simulink model "Modelo_MI_simulink_standalone_ver2020b"  (R2020b)
settings: Solver=ode5  StartTime=0.0  StopTime=tsim  FixedStep=tstep  MaxStep=1e-4  RelTol=1e-3
PreLoadFcn:
  | % Estructura para parametros del motor de induccion
  | 
  | inversor_select = 0;
  | tsim = 20;
  | tstep = 1e-4;
  | 
  | nomvals = struct('Pnom',745.7,'v_Srmsnom',230,'i_Srmsnom',0,'psi_Rmagnom',0,'w_Rnom',180.64,'tau_Rnom',0);
  | elecparams = struct('n_p',2,'R_S',2.516,'R_R',1.941,'L_S',0.234,'L_R',0.2303,'M',0.2226,'sigma',0,'gamma',0);
  | mechparams = struct('J',0.0062764,'b',0.00011);
  | 
  | nomvals.i_Srmsnom = nomvals.Pnom/nomvals.v_Srmsnom;
  | nomvals.psi_Rmagnom = elecparams.M*nomvals.i_Srmsnom/sqrt(2);
  | nomvals.tau_Rnom = nomvals.Pnom/nomvals.w_Rnom;
  | 
  | elecparams.sigma = elecparams.L_S-(elecparams.M^2/elecparams.L_R);
  | elecparams.gamma = (elecparams.R_S*elecparams.L_R^2+elecparams.R_R*elecparams.M^2)/(elecparams.sigma*elecparams.L_R^2);
  | 
  | MI_params = struct('nomvals',nomvals,'elecparams',elecparams,'mechparams',mechparams);
  | 
  | MI_bus_info = Simulink.Bus.createObject(MI_params);
  | MI_bus = evalin('base', MI_bus_info.busName);
libraries: powerlib x16, mcbcontrolslib x4, powerlib_meascontrol x2, simulink x1
settings Model: Creator=HP  LastModifiedBy=HP
settings DebuggingCC: UnconnectedInputMsg=none  UnconnectedOutputMsg=none  UnconnectedLineMsg=none
settings ModelReferenceCC: EnableRefExpFcnMdlSchedulingChecks=off

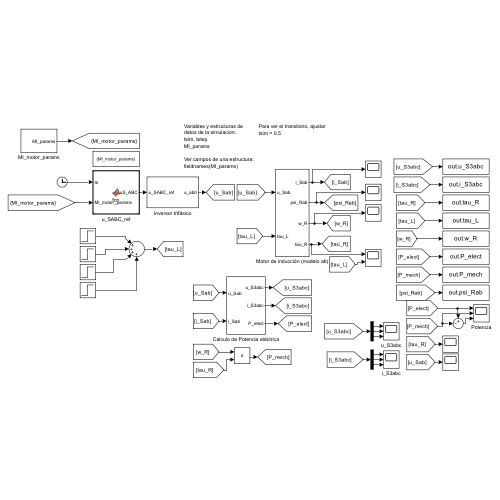
[thumbnail: Simulink's stored preview of the top-level diagram]
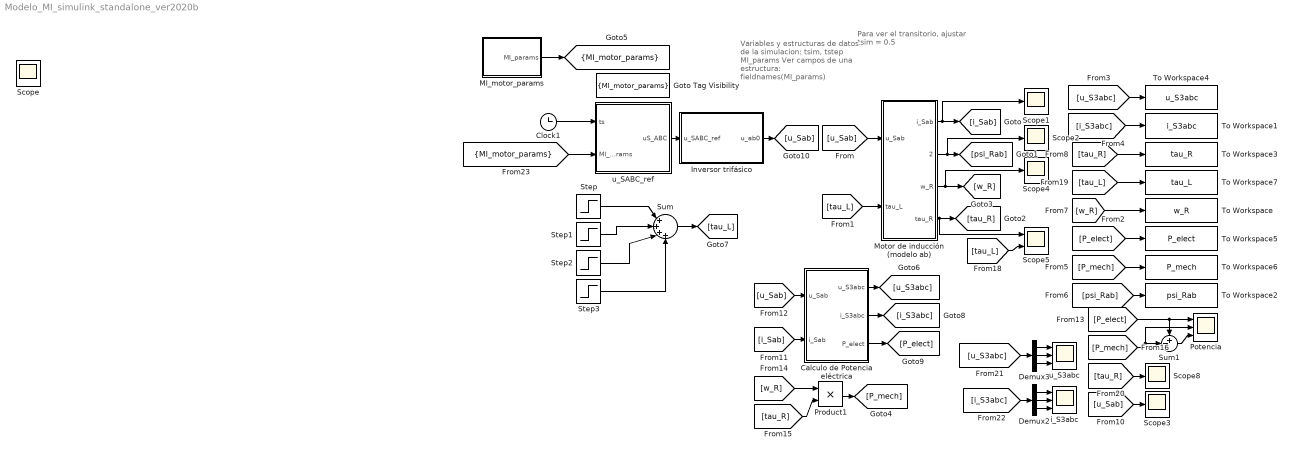
== system Modelo_MI_simulink_standalone_ver2020b ==
  note: Para ver el transitorio, ajustar
      | tsim = 0.5
  note: Variables y estructuras de datos de la simulacion:
      | tsim, tstep
      | MI_params
      |
      | Ver campos de una estructura:
      | fieldnames(MI_params)
  Calculo de Potencia eléctrica : Subsystem
  Clock1 : Clock
  Demux2 : Demux  Outputs=3
  Demux3 : Demux  Outputs=3
  Goto Tag Visibility : GotoTagVisibility  GotoTag=MI_motor_params
  Inversor trifásico : Subsystem
  MI_motor_params : Subsystem
  Motor de inducción (modelo ab) : Subsystem
  Potencia : Scope  NumInputPorts=3
  Product1 : Product
  Scope{,1..4,8} (6 alike) : Scope
  Scope5 : Scope  NumInputPorts=2
  Step : Step  Time=2  After=MI_params.nomvals.tau_Rnom/4  SampleTime=0
  Step1 : Step  Time=4  After=MI_params.nomvals.tau_Rnom/4  SampleTime=0
  Step2 : Step  Time=6  After=MI_params.nomvals.tau_Rnom/4  SampleTime=0
  Step3 : Step  Time=8  After=MI_params.nomvals.tau_Rnom/4  SampleTime=0
  Sum : Sum  Inputs=|++++
  Sum1 : Sum  Inputs=+-|
  To Workspace : ToWorkspace  VariableName=w_R  SaveFormat=Timeseries  SampleTime=-1
  To Workspace1 : ToWorkspace  VariableName=i_S3abc  SaveFormat=Timeseries  SampleTime=-1
  To Workspace2 : ToWorkspace  VariableName=psi_Rab  SaveFormat=Timeseries  SampleTime=-1
  To Workspace3 : ToWorkspace  VariableName=tau_R  SaveFormat=Timeseries  SampleTime=-1
  To Workspace4 : ToWorkspace  VariableName=u_S3abc  SaveFormat=Timeseries  SampleTime=-1
  To Workspace5 : ToWorkspace  VariableName=P_elect  SaveFormat=Timeseries  SampleTime=-1
  To Workspace6 : ToWorkspace  VariableName=P_mech  SaveFormat=Timeseries  SampleTime=-1
  To Workspace7 : ToWorkspace  VariableName=tau_L  SaveFormat=Timeseries  SampleTime=-1
  i_S3abc : Scope  NumInputPorts=3
  u_S3abc : Scope  NumInputPorts=3
  u_SABC_ref : MATLAB Function  TreatAsAtomicUnit=on
  tag scope: MI_motor_params=scoped
  wires:
  [w_R] -> To Workspace/1
  [i_S3abc] -> To Workspace1/1
  [tau_R] -> To Workspace3/1
  Step/1 -> Sum/1
  Step1/1 -> Sum/2
  Step2/1 -> Sum/3
  Step3/1 -> Sum/4
  Sum/1 -> [tau_L]
  [i_Sab] -> Calculo de Potencia eléctrica/2(i_Sab)
  Calculo de Potencia eléctrica/3(P_elect) -> [P_elect]
  Calculo de Potencia eléctrica/1(u_S3abc) -> [u_S3abc]
  [u_Sab] -> Calculo de Potencia eléctrica/1(u_Sab)
  Calculo de Potencia eléctrica/2(i_S3abc) -> [i_S3abc]
  [tau_L] -> Scope5/2
  Motor de inducción (modelo ab)/2(psi_Rab) -> Scope2/1, [psi_Rab]
  Motor de inducción (modelo ab)/1(i_Sab) -> Scope1/1, [i_Sab]
  Motor de inducción (modelo ab)/4(tau_R) -> Scope5/1, [tau_R]
  Motor de inducción (modelo ab)/3(w_R) -> [w_R], Scope4/1
  [u_Sab] -> Motor de inducción (modelo ab)/1(u_Sab)
  [tau_L] -> Motor de inducción (modelo ab)/2(tau_L)
  [u_S3abc] -> To Workspace4/1
  Demux3/3 -> u_S3abc/3
  Demux2/3 -> i_S3abc/3
  Demux3/1 -> u_S3abc/1
  Demux2/1 -> i_S3abc/1
  Demux3/2 -> u_S3abc/2
  Demux2/2 -> i_S3abc/2
  [P_elect] -> To Workspace5/1
  [P_mech] -> To Workspace6/1
  [tau_L] -> To Workspace7/1
  [MI_motor_params] -> u_SABC_ref/2(MI_motor_params)
  Clock1/1 -> u_SABC_ref/1(ts)
  [psi_Rab] -> To Workspace2/1
  [u_Sab] -> Scope3/1
  u_SABC_ref/1(uS_ABC) -> Inversor trifásico/1(u_SABC_ref)
  Inversor trifásico/1(u_ab0) -> [u_Sab]
  [tau_R] -> Scope8/1
  [P_elect] -> Potencia/1, Sum1/1
  [tau_R] -> Product1/2
  [P_mech] -> Potencia/2, Sum1/2
  Product1/1 -> [P_mech]
  Sum1/1 -> Potencia/3
  [w_R] -> Product1/1
  [u_S3abc] -> Demux3/1
  [i_S3abc] -> Demux2/1
  MI_motor_params/1(MI_params) -> [MI_motor_params]

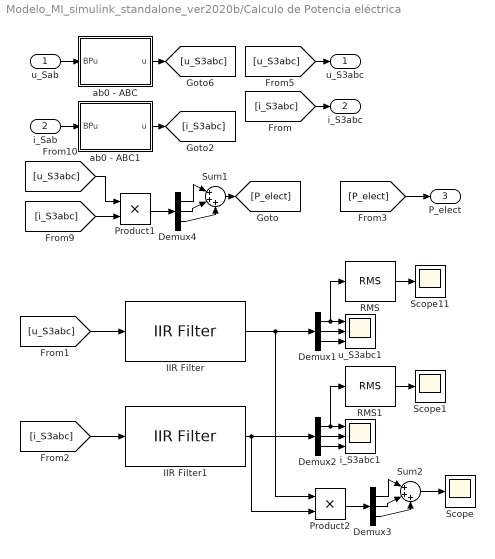
== system Modelo_MI_simulink_standalone_ver2020b/Calculo de Potencia eléctrica ==
  u_Sab : Inport
  i_Sab : Inport  Port=2
  Demux{1..4} (4 alike) : Demux  Outputs=3
  IIR Filter : mcbcontrolslib/IIR Filter  VariantControl=Low Pass Filter  VariantSelect=Low-pass  Filter_constant=0.04  advancedSettings=on  Ts=50e-6  cutOff_freq=132.6291
  IIR Filter1 : mcbcontrolslib/IIR Filter  VariantControl=Low Pass Filter  VariantSelect=Low-pass  Filter_constant=0.04  advancedSettings=on  Ts=50e-6  cutOff_freq=132.6291
  Product1 : Product
  Product2 : Product
  RMS : powerlib_meascontrol/Measurements/RMS  TrueRMS=on  Freq=60  RMSInit=120  Ts=0
  RMS1 : powerlib_meascontrol/Measurements/RMS  TrueRMS=on  Freq=60  RMSInit=120  Ts=0
  Scope : Scope
  Scope1 : Scope
  Scope11 : Scope
  Sum1 : Sum  Inputs=|+++
  Sum2 : Sum  Inputs=|+++
  ab0 - ABC : MATLAB Function  TreatAsAtomicUnit=on
  ab0 - ABC1 : MATLAB Function  TreatAsAtomicUnit=on
  i_S3abc1 : Scope  NumInputPorts=3
  u_S3abc1 : Scope  NumInputPorts=3
  u_S3abc : Outport
  i_S3abc : Outport  Port=2
  P_elect : Outport  Port=3
  wires:
  Demux4/1 -> Sum1/1
  [i_S3abc] -> Product1/2
  i_Sab/1 -> ab0 - ABC1/1(BPu)
  Demux4/3 -> Sum1/3
  [u_S3abc] -> Product1/1
  Demux4/2 -> Sum1/2
  Product1/1 -> Demux4/1
  u_Sab/1 -> ab0 - ABC/1(BPu)
  [u_S3abc] -> u_S3abc/1
  [i_S3abc] -> i_S3abc/1
  ab0 - ABC/1(u) -> [u_S3abc]
  ab0 - ABC1/1(u) -> [i_S3abc]
  IIR Filter/1 -> Product2/1, Demux1/1
  RMS/1 -> Scope11/1
  Demux1/2 -> u_S3abc1/2
  Demux1/3 -> u_S3abc1/3
  Demux1/1 -> RMS/1, u_S3abc1/1
  [u_S3abc] -> IIR Filter/1
  Demux2/1 -> RMS1/1, i_S3abc1/1
  RMS1/1 -> Scope1/1
  Demux2/2 -> i_S3abc1/2
  IIR Filter1/1 -> Product2/2, Demux2/1
  [i_S3abc] -> IIR Filter1/1
  Demux2/3 -> i_S3abc1/3
  Demux3/2 -> Sum2/2
  Demux3/3 -> Sum2/3
  Sum2/1 -> Scope/1
  Product2/1 -> Demux3/1
  Demux3/1 -> Sum2/1
  Sum1/1 -> [P_elect]
  [P_elect] -> P_elect/1

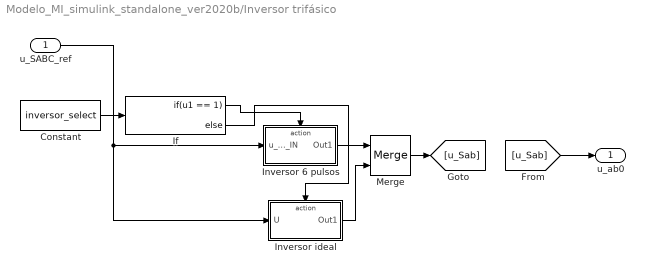
== system Modelo_MI_simulink_standalone_ver2020b/Inversor trifásico ==
  u_SABC_ref : Inport
  Constant : Constant  Value=inversor_select
  If : If  IfExpression=u1 == 1
  Inversor 6 pulsos : Subsystem  TreatAsAtomicUnit=on
  Inversor ideal : Subsystem  TreatAsAtomicUnit=on
  Merge : Merge
  u_ab0 : Outport
  wires:
  [u_Sab] -> u_ab0/1
  If/1 -> Inversor 6 pulsos/Action
  If/2 -> Inversor ideal/Action
  Inversor 6 pulsos/1(Out1) -> Merge/1
  Inversor ideal/1(Out1) -> Merge/2
  Merge/1 -> [u_Sab]
  Constant/1 -> If/1
  u_SABC_ref/1 -> Inversor ideal/1(U), Inversor 6 pulsos/1(u_SABC_IN)

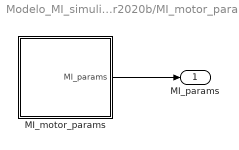
== system Modelo_MI_simulink_standalone_ver2020b/MI_motor_params ==
  MI_motor_params : MATLAB Function  TreatAsAtomicUnit=on
  MI_params : Outport
  wires:
  MI_motor_params/1(MI_params) -> MI_params/1

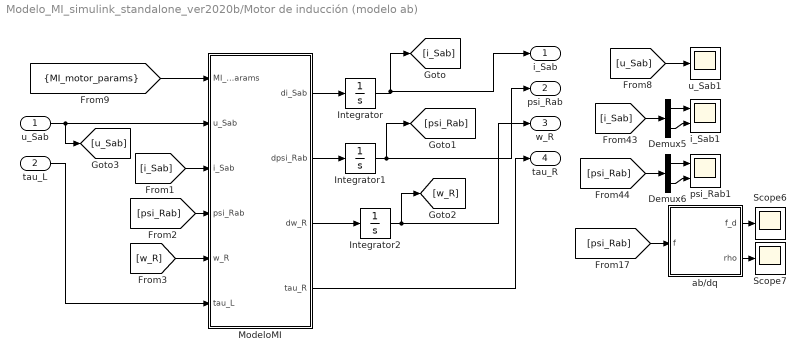
== system Modelo_MI_simulink_standalone_ver2020b/Motor de inducción (modelo ab) ==
  u_Sab : Inport
  tau_L : Inport  Port=2
  Demux5 : Demux  Outputs=2
  Demux6 : Demux  Outputs=2
  Integrator : Integrator
  Integrator1 : Integrator
  Integrator2 : Integrator
  ModeloMI : MATLAB Function  TreatAsAtomicUnit=on
  Scope6 : Scope
  Scope7 : Scope
  ab/dq : MATLAB Function  TreatAsAtomicUnit=on
  i_Sab1 : Scope  NumInputPorts=2
  psi_Rab1 : Scope  NumInputPorts=2
  u_Sab1 : Scope
  i_Sab : Outport
  psi_Rab : Outport  Port=2
  w_R : Outport  Port=3
  tau_R : Outport  Port=4
  wires:
  ModeloMI/3(dw_R) -> Integrator2/1
  [i_Sab] -> ModeloMI/3(i_Sab)
  [MI_motor_params] -> ModeloMI/1(MI_motor_params)
  [psi_Rab] -> ModeloMI/4(psi_Rab)
  [w_R] -> ModeloMI/5(w_R)
  Integrator2/1 -> w_R/1, [w_R]
  ModeloMI/2(dpsi_Rab) -> Integrator1/1
  tau_L/1 -> ModeloMI/6(tau_L)
  ModeloMI/1(di_Sab) -> Integrator/1
  u_Sab/1 -> ModeloMI/2(u_Sab), [u_Sab]
  ModeloMI/4(tau_R) -> tau_R/1
  Integrator/1 -> [i_Sab], i_Sab/1
  Integrator1/1 -> [psi_Rab], psi_Rab/1
  [psi_Rab] -> ab/dq/1(f)
  ab/dq/2(rho) -> Scope7/1
  Demux6/2 -> psi_Rab1/2
  Demux5/2 -> i_Sab1/2
  [u_Sab] -> u_Sab1/1
  Demux6/1 -> psi_Rab1/1
  [psi_Rab] -> Demux6/1
  Demux5/1 -> i_Sab1/1
  [i_Sab] -> Demux5/1
  ab/dq/1(f_d) -> Scope6/1

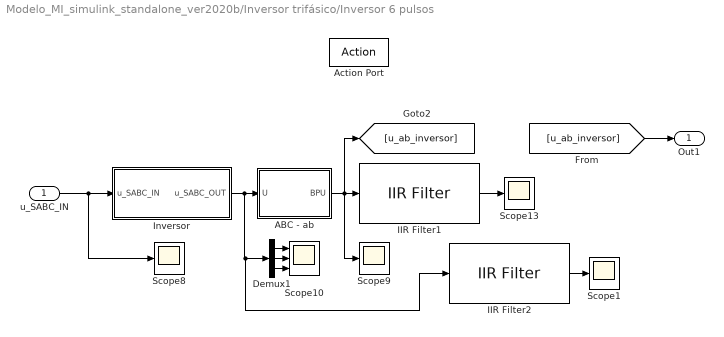
== system Modelo_MI_simulink_standalone_ver2020b/Inversor trifásico/Inversor 6 pulsos ==
  u_SABC_IN : Inport
  Action Port : ActionPort  ActionPortLabel=if(u1 == 1)
  ABC - ab : MATLAB Function  TreatAsAtomicUnit=on
  Demux1 : Demux  Outputs=3
  IIR Filter1 : mcbcontrolslib/IIR Filter  VariantControl=Low Pass Filter  VariantSelect=Low-pass  Filter_constant=0.04  advancedSettings=on  Ts=50e-6  cutOff_freq=132.6291
  IIR Filter2 : mcbcontrolslib/IIR Filter  VariantControl=Low Pass Filter  VariantSelect=Low-pass  Filter_constant=0.04  advancedSettings=on  Ts=50e-6  cutOff_freq=132.6291
  Inversor : Subsystem
  Scope{1,8..9,13} (4 alike) : Scope
  Scope10 : Scope  NumInputPorts=3
  Out1 : Outport
  wires:
  IIR Filter2/1 -> Scope1/1
  ABC - ab/1(BPU) -> [u_ab_inversor], IIR Filter1/1, Scope9/1
  Demux1/3 -> Scope10/3
  Inversor/1(u_SABC_OUT) -> IIR Filter2/1, Demux1/1, ABC - ab/1(U)
  Demux1/1 -> Scope10/1
  Demux1/2 -> Scope10/2
  IIR Filter1/1 -> Scope13/1
  u_SABC_IN/1 -> Scope8/1, Inversor/1(u_SABC_IN)
  [u_ab_inversor] -> Out1/1

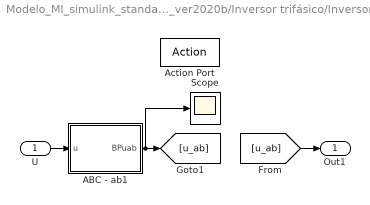
== system Modelo_MI_simulink_standalone_ver2020b/Inversor trifásico/Inversor ideal ==
  U : Inport
  Action Port : ActionPort  ActionPortLabel=else
  ABC - ab1 : MATLAB Function  TreatAsAtomicUnit=on
  Scope : Scope
  Out1 : Outport
  wires:
  ABC - ab1/1(BPuab) -> Scope/1, [u_ab]
  U/1 -> ABC - ab1/1(u)
  [u_ab] -> Out1/1

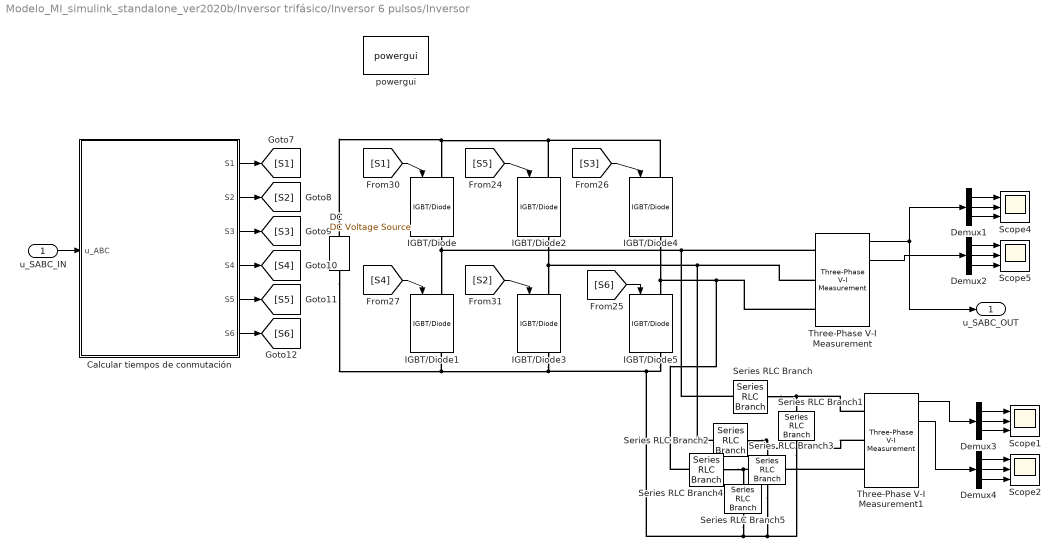
== system Modelo_MI_simulink_standalone_ver2020b/Inversor trifásico/Inversor 6 pulsos/Inversor ==
  u_SABC_IN : Inport
  Calcular tiempos de conmutación : Subsystem
  "DC " : powerlib/Electrical Sources/DC Voltage Source  Amplitude=310  Measurements=None
  Demux{1..4} (4 alike) : Demux  Outputs=3
  IGBT/Diode{,1..5} (6 alike) : powerlib/Power Electronics/IGBT//Diode  Ron=1e-3  Rs=1e5  Cs=inf  Measurements=on
  Scope{1..2,4..5} (4 alike) : Scope  NumInputPorts=3
  Series RLC Branch : powerlib/Elements/Series RLC Branch  LConnTagsString=__new0  RConnTagsString=__new0  BranchType=R  Resistance=1  Inductance=1e-3  SetiL0=off  InitialCurrent=0  Capacitance=1e-6  Setx0=off  InitialVoltage=0  Measurements=None
  Series RLC Branch1 : powerlib/Elements/Series RLC Branch  LConnTagsString=__new0  RConnTagsString=__new0  BranchType=C  Resistance=1  Inductance=1e-3  SetiL0=off  InitialCurrent=0  Capacitance=120e-6  Setx0=off  InitialVoltage=0  Measurements=None
  Series RLC Branch2 : powerlib/Elements/Series RLC Branch  LConnTagsString=__new0  RConnTagsString=__new0  BranchType=R  Resistance=1  Inductance=1e-3  SetiL0=off  InitialCurrent=0  Capacitance=1e-6  Setx0=off  InitialVoltage=0  Measurements=None
  Series RLC Branch3 : powerlib/Elements/Series RLC Branch  LConnTagsString=__new0  RConnTagsString=__new0  BranchType=C  Resistance=1  Inductance=1e-3  SetiL0=off  InitialCurrent=0  Capacitance=120e-6  Setx0=off  InitialVoltage=0  Measurements=None
  Series RLC Branch4 : powerlib/Elements/Series RLC Branch  LConnTagsString=__new0  RConnTagsString=__new0  BranchType=R  Resistance=1  Inductance=1e-3  SetiL0=off  InitialCurrent=0  Capacitance=1e-6  Setx0=off  InitialVoltage=0  Measurements=None
  Series RLC Branch5 : powerlib/Elements/Series RLC Branch  LConnTagsString=__new0  RConnTagsString=__new0  BranchType=C  Resistance=1  Inductance=1e-3  SetiL0=off  InitialCurrent=0  Capacitance=120e-6  Setx0=off  InitialVoltage=0  Measurements=None
  Three-Phase V-I Measurement : powerlib/Measurements/Three-Phase V-I Measurement  VoltageMeasurement=phase-to-phase  SetLabelV=off  LabelV=Vabc  Vpu=off  VpuLL=off  CurrentMeasurement=yes  SetLabelI=off  LabelI=Iabc  Ipu=off  Pbase=100e6  Vbase=500e3  OutputType=Complex  PhasorSimulation=off  PSBequivalent=0
  Three-Phase V-I Measurement1 : powerlib/Measurements/Three-Phase V-I Measurement  VoltageMeasurement=phase-to-phase  SetLabelV=off  LabelV=Vabc  Vpu=off  VpuLL=off  CurrentMeasurement=yes  SetLabelI=off  LabelI=Iabc  Ipu=off  Pbase=100e6  Vbase=500e3  OutputType=Complex  PhasorSimulation=off  PSBequivalent=0
  powergui : powerlib/powergui  Priority=1  SimulationMode=Continuous  SampleTime=10e-6  frequency=60  Iterations=50  frequencyindice=0  Pbase=100e6  ErrMax=1e-4  UnitsV=kV  UnitsW=MW  buscounter=0  FunctionMessages=off  echomessages=off  EnableUseOfTLC=off  CurrentSourceSwitches=on  DisableSnubberDevices=off  DisableRonSwitches=off  DisableVfSwitches=off  DisplayEquations=off  AutomaticDiscreteSolvers=off  SolverType=Tustin/Backward Euler (TBE)  Interpol=off  ExternalGateDelay=off  methode=off  Ts=10  x0status=blocks  SPID=off  SwTol=0  HookPort=off  NonlinearTolerance=1e-4  nMaxIteration=100  ContinueOnMaxIteration=off  RestoreLinks=warning  ResistiveCurrentMeasurement=off  Frange=[0:2:500]  Ylog=off  Xlog=on  ShowGrid=off  save=off  variable=ZData  structure=ScopeData1  ZoomFFT=off  StartTime=0.0  cycles=1  DisplayStyle=1  fundamental=50  FreqAxis=off  MaxFrequency=1000  frequencyindicesteady=1  RmsSteady=1  display=off
  u_SABC_OUT : Outport
  wires:
  [S5] -> IGBT/Diode2/1
  Demux2/3 -> Scope5/3
  Demux2/2 -> Scope5/2
  Three-Phase V-I Measurement/1 -> Demux1/1, u_SABC_OUT/1
  Demux1/2 -> Scope4/2
  Demux2/1 -> Scope5/1
  Demux1/1 -> Scope4/1
  Calcular tiempos de conmutación/5(S5) -> [S5]
  Three-Phase V-I Measurement/2 -> Demux2/1
  u_SABC_IN/1 -> Calcular tiempos de conmutación/1(u_ABC)
  [S3] -> IGBT/Diode4/1
  Calcular tiempos de conmutación/2(S2) -> [S2]
  Calcular tiempos de conmutación/6(S6) -> [S6]
  Calcular tiempos de conmutación/4(S4) -> [S4]
  [S1] -> IGBT/Diode/1
  Calcular tiempos de conmutación/3(S3) -> [S3]
  Calcular tiempos de conmutación/1(S1) -> [S1]
  Demux1/3 -> Scope4/3
  [S2] -> IGBT/Diode3/1
  [S6] -> IGBT/Diode5/1
  [S4] -> IGBT/Diode1/1
  Three-Phase V-I Measurement1/2 -> Demux4/1
  Three-Phase V-I Measurement1/1 -> Demux3/1
  Demux4/1 -> Scope2/1
  Demux3/1 -> Scope1/1
  Demux4/2 -> Scope2/2
  Demux3/3 -> Scope1/3
  Demux3/2 -> Scope1/2
  Demux4/3 -> Scope2/3
  connections:
  IGBT/Diode5/LConn1 -- Series RLC Branch4/LConn1 -- Three-Phase V-I Measurement/LConn3 -- IGBT/Diode4/RConn1
  IGBT/Diode2/RConn1 -- Three-Phase V-I Measurement/LConn2 -- Series RLC Branch2/LConn1 -- IGBT/Diode3/LConn1
  "DC "/RConn1 -- IGBT/Diode/LConn1 -- IGBT/Diode4/LConn1 -- IGBT/Diode2/LConn1
  IGBT/Diode/RConn1 -- Series RLC Branch/LConn1 -- Three-Phase V-I Measurement/LConn1 -- IGBT/Diode1/LConn1
  Series RLC Branch/RConn1 -- Three-Phase V-I Measurement1/LConn1 -- Series RLC Branch1/LConn1
  IGBT/Diode3/RConn1 -- Series RLC Branch1/RConn1 -- Series RLC Branch3/RConn1 -- Series RLC Branch5/RConn1 -- IGBT/Diode5/RConn1 -- "DC "/LConn1 -- IGBT/Diode1/RConn1
  Series RLC Branch2/RConn1 -- Three-Phase V-I Measurement1/LConn2 -- Series RLC Branch3/LConn1
  Series RLC Branch4/RConn1 -- Three-Phase V-I Measurement1/LConn3 -- Series RLC Branch5/LConn1

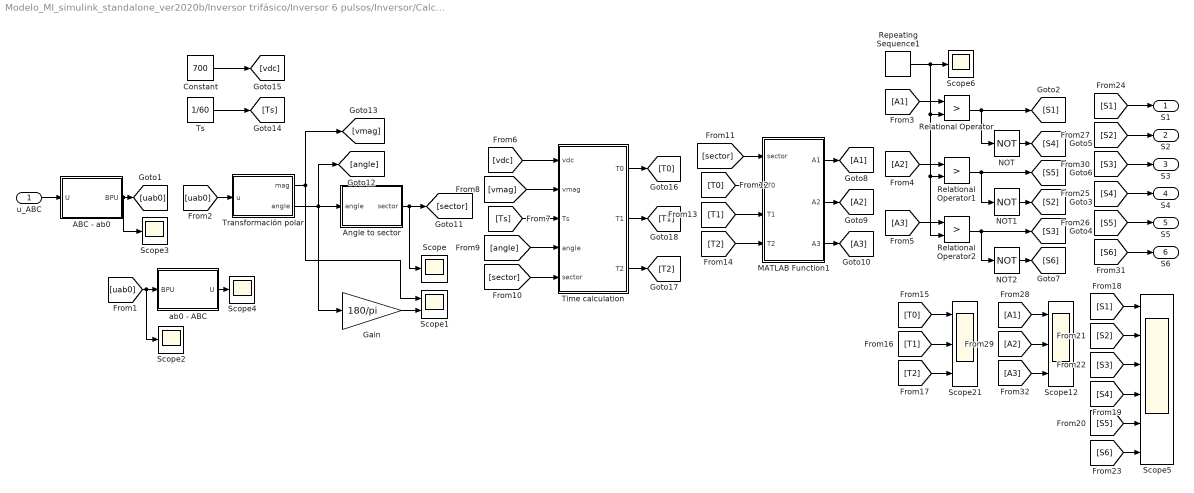
== system Modelo_MI_simulink_standalone_ver2020b/Inversor trifásico/Inversor 6 pulsos/Inversor/Calcular tiempos de conmutación ==
  u_ABC : Inport
  ABC - ab0 : MATLAB Function  TreatAsAtomicUnit=on
  Angle to sector : MATLAB Function  TreatAsAtomicUnit=on
  Constant : Constant  Value=700
  Gain : Gain  Gain=180/pi
  MATLAB Function1 : MATLAB Function  TreatAsAtomicUnit=on
  NOT : Logic  Operator=NOT  IconShape=distinctive  AllPortsSameDT=off  OutDataTypeStr=boolean
  NOT1 : Logic  Operator=NOT  IconShape=distinctive  AllPortsSameDT=off  OutDataTypeStr=boolean
  NOT2 : Logic  Operator=NOT  IconShape=distinctive  AllPortsSameDT=off  OutDataTypeStr=boolean
  Relational Operator : RelationalOperator  Operator=>  OutDataTypeStr=boolean  RndMeth=Nearest
  Relational Operator1 : RelationalOperator  Operator=>  OutDataTypeStr=boolean  RndMeth=Nearest
  Relational Operator2 : RelationalOperator  Operator=>  OutDataTypeStr=boolean  RndMeth=Nearest
  Repeating Sequence1 : simulink/Sources/Repeating Sequence  rep_seq_t=[0 1]*[1/5000]  rep_seq_y=[0 1/60]
  Scope{,2..4,6} (5 alike) : Scope
  Scope1 : Scope  NumInputPorts=2
  Scope12 : Scope  NumInputPorts=3
  Scope21 : Scope  NumInputPorts=3
  Scope5 : Scope  NumInputPorts=6
  Time calculation : MATLAB Function  TreatAsAtomicUnit=on
  Transformación polar : MATLAB Function  TreatAsAtomicUnit=on
  Ts : Constant  Value=1/60
  ab0 - ABC : MATLAB Function  TreatAsAtomicUnit=on
  S1 : Outport
  S2 : Outport  Port=2
  S3 : Outport  Port=3
  S4 : Outport  Port=4
  S5 : Outport  Port=5
  S6 : Outport  Port=6
  wires:
  [vmag] -> Time calculation/2(vmag)
  [sector] -> Time calculation/5(sector)
  Relational Operator2/1 -> NOT2/1, [S3]
  [Ts] -> Time calculation/3(Ts)
  NOT2/1 -> [S6]
  [S6] -> Scope5/6
  Transformación polar/1(mag) -> [vmag], Scope1/1
  [T1] -> Scope21/2
  [S3] -> Scope5/3
  Time calculation/3(T2) -> [T2]
  [T2] -> Scope21/3
  [T1] -> MATLAB Function1/3(T1)
  [uab0] -> Transformación polar/1(u)
  Time calculation/2(T1) -> [T1]
  Relational Operator1/1 -> NOT1/1, [S5]
  NOT1/1 -> [S2]
  Angle to sector/1(sector) -> [sector], Scope/1
  [S1] -> Scope5/1
  [uab0] -> Scope2/1, ab0 - ABC/1(BPU)
  [angle] -> Time calculation/4(angle)
  [S4] -> Scope5/4
  [A2] -> Relational Operator1/1
  MATLAB Function1/2(A2) -> [A2]
  NOT/1 -> [S4]
  [T2] -> MATLAB Function1/4(T2)
  Transformación polar/2(angle) -> [angle], Gain/1, Angle to sector/1(angle)
  MATLAB Function1/1(A1) -> [A1]
  Gain/1 -> Scope1/2
  Relational Operator/1 -> NOT/1, [S1]
  [A3] -> Scope12/3
  ab0 - ABC/1(U) -> Scope4/1
  Repeating Sequence1/1 -> Scope6/1, Relational Operator2/2, Relational Operator1/2, Relational Operator/2
  Constant/1 -> [vdc]
  [S2] -> Scope5/2
  MATLAB Function1/3(A3) -> [A3]
  [T0] -> Scope21/1
  [S5] -> Scope5/5
  [A1] -> Relational Operator/1
  [T0] -> MATLAB Function1/2(T0)
  [vdc] -> Time calculation/1(vdc)
  [sector] -> MATLAB Function1/1(sector)
  Ts/1 -> [Ts]
  [A3] -> Relational Operator2/1
  Time calculation/1(T0) -> [T0]
  [A1] -> Scope12/1
  [A2] -> Scope12/2
  [S6] -> S6/1
  [S5] -> S5/1
  [S4] -> S4/1
  [S3] -> S3/1
  [S2] -> S2/1
  [S1] -> S1/1
  u_ABC/1 -> ABC - ab0/1(U)
  ABC - ab0/1(BPU) -> Scope3/1, [uab0]

== matlab function Modelo_MI_simulink_standalone_ver2020b/Inversor trifásico/Inversor 6 pulsos/Inversor/Calcular tiempos de conmutación/MATLAB Function1 ==
  data: sector input; A1 output; T0 input; T1 input; T2 input; A2 output; A3 output
function [A1,A2,A3] = fcn(sector,T0,T1,T2)

a = T0/2;
b = T1 + T0/2;
c = T2 + T0/2;
d = T1 + T2 + T0/2;

switch sector
    case 1
        A1 = d;
        A2 = c;
        A3 = a;
    case 2
        A1 = b;
        A2 = d;
        A3 = a;
    case 3
        A1 = a;
        A2 = d;
        A3 = c;
    case 4
        A1 = a;
        A2 = b;
        A3 = d;
    case 5
        A1 = c;
        A2 = a;
        A3 = d;
    case 6
        A1 = d;
        A2 = a;
        A3 = b;
    otherwise
        A1 = -1;
        A2 = -1;
        A3 = -1;
end

%A = [A1;A2;A3];

== matlab function Modelo_MI_simulink_standalone_ver2020b/Inversor trifásico/Inversor 6 pulsos/Inversor/Calcular tiempos de conmutación/Time calculation ==
  data: vdc input; vmag input; T0 output; Ts input; angle input; sector input; T1 output; T2 output
function [T0,T1,T2] = fcn(vdc,vmag,Ts,angle,sector)

a = sqrt(3)*vmag/vdc*Ts;

T1 = a*sin(sector*pi/3 - angle);
T2 = a*sin(-(sector-1)*pi/3 + angle);

T0 = Ts - T1 - T2;

== matlab function Modelo_MI_simulink_standalone_ver2020b/Inversor trifásico/Inversor 6 pulsos/Inversor/Calcular tiempos de conmutación/Transformación polar ==
  data: u input; mag output; angle output
function [mag,angle] = fcn(u)

% u_alpha = u(1);
% u_beta = u(2);
%u_zeta = u(3);

[mag,angle] = Polar_transform(u);

function [mag,angle] = Polar_transform(u)
u1 = u(1);
u2 = u(2);

mag = sqrt(u1^2+u2^2);
angle = atan2(u2,u1);

== matlab function Modelo_MI_simulink_standalone_ver2020b/Inversor trifásico/Inversor 6 pulsos/Inversor/Calcular tiempos de conmutación/ab0 - ABC ==
  data: BPU input size=[3,1]; U output size=[3,1]
function U = fcn(BPU)

BP = 2/3*[1,-1/2,-1/2;
          0,sqrt(3)/2,-sqrt(3)/2;
          1/2,1/2,1/2];

% Power invariant
% BP = sqrt(2/3)*[1,-1/2,-1/2;
%                 0,sqrt(3)/2,-sqrt(3)/2
%                 1/sqrt(2),1/sqrt(2),1/sqrt(2)];

U = BP^-1*BPU;

== matlab function Modelo_MI_simulink_standalone_ver2020b/Inversor trifásico/Inversor 6 pulsos/ABC - ab ==
  data: U input size=[3,1]; BPU output size=[2,1]
function BPU = fcn(U)

% BP = 2/3*[1,-1/2,-1/2;
%           0,sqrt(3)/2,-sqrt(3)/2];
%           %1/2,1/2,1/2];

% Power invariant
BP = sqrt(2/3)*[1,-1/2,-1/2;
                0,sqrt(3)/2,-sqrt(3)/2];
                %1/sqrt(2),1/sqrt(2),1/sqrt(2)];

BPU = BP*U;

== matlab function Modelo_MI_simulink_standalone_ver2020b/Inversor trifásico/Inversor ideal/ABC - ab1 ==
  data: u input size=[3,1]; BPuab output size=[2,1]
function BPuab = fcn(u)

% Power invariant
BP = Clarke_transform(1);

BPu = BP*u;

BPuab = [BPu(1);BPu(2)];

function BP = Clarke_transform(opt_power_invariant)
if opt_power_invariant == 0
    BP = 2/3*[1,-1/2,-1/2;
              0,sqrt(3)/2,-sqrt(3)/2;
              1/2,1/2,1/2];
else
    % Power invariant
    BP = sqrt(2/3)*[1,-1/2,-1/2;
                    0,sqrt(3)/2,-sqrt(3)/2;
                    1/sqrt(2),1/sqrt(2),1/sqrt(2)];
end

== matlab function Modelo_MI_simulink_standalone_ver2020b/Motor de inducción (modelo ab)/ModeloMI ==
  data: MI_motor_params input Bus: MI_bus; di_Sab output double size=[2 1]; dpsi_Rab output double size=[2 1]; dw_R output size=1; u_Sab input double size=[2 1]; i_Sab input double size=[2 1]; psi_Rab input double size=[2 1]; w_R input double size=1; tau_R output size=1; tau_L input
function [di_Sab,dpsi_Rab,dw_R,tau_R] = fcn(MI_motor_params,u_Sab,i_Sab,psi_Rab,w_R,tau_L)

% [di_Sab,dpsi_Rab,dw_R,tau_R] = MI_model.MI_space_state(MI_motor_params,u_Sab,i_Sab,psi_Rab,w_R,tau_L);

%R_S = MI_motor_params.elecparams.R_S;
R_R = MI_motor_params.elecparams.R_R;
%L_S = MI_motor_params.elecparams.L_S;
L_R = MI_motor_params.elecparams.L_R;
M = MI_motor_params.elecparams.M;
n_p = MI_motor_params.elecparams.n_p;

J = MI_motor_params.mechparams.J;
b = MI_motor_params.mechparams.b;

sigma = MI_motor_params.elecparams.sigma;
gamma = MI_motor_params.elecparams.gamma;
% sigma = L_S - M^2/L_R;
% gamma = M^2*R_R/(sigma*L_R^2)+R_S/sigma;


u_Sa = u_Sab(1);
u_Sb = u_Sab(2);

i_Sa = i_Sab(1);
i_Sb = i_Sab(2);

psi_Ra = psi_Rab(1);
psi_Rb = psi_Rab(2);

tau_R = n_p*M/L_R*(i_Sb*psi_Ra-i_Sa*psi_Rb);

x = [i_Sa;i_Sb;psi_Ra;psi_Rb];

A = [-gamma      , 0            , (M*R_R)/(sigma*L_R^2)    , (n_p*M)/(sigma*L_R)*w_R ;
     0           , -gamma       , -(n_p*M)/(sigma*L_R)*w_R , (M*R_R)/(sigma*L_R^2)   ; 
     (R_R*M)/L_R , 0            , -R_R/L_R                 , -n_p*w_R                ;
     0           , (R_R*M)/L_R  , n_p*w_R                  , -R_R/L_R                ];

B = [1/sigma , 0       ;
     0       , 1/sigma ;
     0       , 0       ;
     0       , 0       ];

dx = A*x + B*[u_Sa;u_Sb];

di_Sab = dx(1:2);
dpsi_Rab = dx(3:4);

dw_R = (1/J)*tau_R - (b/J)*w_R - (1/J)*tau_L;

== matlab function Modelo_MI_simulink_standalone_ver2020b/Inversor trifásico/Inversor 6 pulsos/Inversor/Calcular tiempos de conmutación/ABC - ab0 ==
  data: U input size=[3,1]; BPU output size=[3,1]
function BPU = fcn(U)

BP = 2/3*[1,-1/2,-1/2;
          0,sqrt(3)/2,-sqrt(3)/2;
          1/2,1/2,1/2];

% Power invariant
% BP = sqrt(2/3)*[1,-1/2,-1/2;
%                 0,sqrt(3)/2,-sqrt(3)/2
%                 1/sqrt(2),1/sqrt(2),1/sqrt(2)];

BPU = BP*U;

== matlab function Modelo_MI_simulink_standalone_ver2020b/Calculo de Potencia eléctrica/ab0 - ABC ==
  data: BPu input size=[2,1]; u output size=[3,1]
function u = fcn(BPu)

BPu = vertcat(BPu,0);

% Power invariant
BP = Clarke_transform(1);

u = BP^-1*BPu;

function BP = Clarke_transform(opt_power_invariant)
if opt_power_invariant == 0
    BP = 2/3*[1,-1/2,-1/2;
              0,sqrt(3)/2,-sqrt(3)/2;
              1/2,1/2,1/2];
else
    % Power invariant
    BP = sqrt(2/3)*[1,-1/2,-1/2;
                    0,sqrt(3)/2,-sqrt(3)/2;
                    1/sqrt(2),1/sqrt(2),1/sqrt(2)];
end

== matlab function Modelo_MI_simulink_standalone_ver2020b/u_SABC_ref ==
  data: ts input; uS_ABC output size=[3,1]; MI_motor_params input
function uS_ABC = fcn(ts,MI_motor_params)

V_Srmsnom = MI_motor_params.nomvals.v_Srmsnom; % Vrms L-L

ws = 2*pi*60; %rad/s
Vmax = V_Srmsnom*sqrt(2/3); %Vpico L-N

uS_A = Vmax*sin(ws*ts);
uS_B = Vmax*sin(ws*ts+4*pi/3);
uS_C = Vmax*sin(ws*ts+2*pi/3);

uS_ABC = [uS_A;uS_B;uS_C];

== matlab function Modelo_MI_simulink_standalone_ver2020b/Calculo de Potencia eléctrica/ab0 - ABC1 ==
  data: BPu input size=[2,1]; u output size=[3,1]
function u = fcn(BPu)

BPu = vertcat(BPu,0);

% Power invariant
BP = Clarke_transform(1);

u = BP^-1*BPu;

function BP = Clarke_transform(opt_power_invariant)
if opt_power_invariant == 0
    BP = 2/3*[1,-1/2,-1/2;
              0,sqrt(3)/2,-sqrt(3)/2;
              1/2,1/2,1/2];
else
    % Power invariant
    BP = sqrt(2/3)*[1,-1/2,-1/2;
                    0,sqrt(3)/2,-sqrt(3)/2;
                    1/sqrt(2),1/sqrt(2),1/sqrt(2)];
end

== matlab function Modelo_MI_simulink_standalone_ver2020b/Motor de inducción (modelo ab)/ab//dq ==
  data: f input; f_d output; rho output
function [f_d,rho] = fcn(f)

[f_d,rho] = Polar_transform(f);

function [mag,angle] = Polar_transform(u)
u1 = u(1);
u2 = u(2);

mag = sqrt(u1^2+u2^2);
angle = atan2(u2,u1);

== matlab function Modelo_MI_simulink_standalone_ver2020b/MI_motor_params/MI_motor_params ==
  data: MI_params output Bus: MI_bus
function MI_params = fcn()


% MI 0.4 hp
%300,380,361.283,1,15.6,23.2,1.44,1.5,1.42,0.000711,0.00014

% MI 1hp
%745.7,230,180.64,2,2.516,1.9461,0.234,0.2303,0.2226,0.0062764,0.00011

% MI 5hp
%3728.5,460,183.2595,2,1.115,1.083,0.20967,0.20967,0.2037,0.02,0.005752

nomvals = struct('Pnom',745.7,'v_Srmsnom',230,'i_Srmsnom',0,'psi_Rmagnom',0,'w_Rnom',180.64,'tau_Rnom',0);
elecparams = struct('n_p',2,'R_S',2.516,'R_R',1.941,'L_S',0.234,'L_R',0.2303,'M',0.2226,'sigma',0,'gamma',0);
mechparams = struct('J',0.0062764,'b',0.00011);

nomvals.i_Srmsnom = nomvals.Pnom/nomvals.v_Srmsnom;
nomvals.psi_Rmagnom = elecparams.M*nomvals.i_Srmsnom/sqrt(2);
nomvals.tau_Rnom = nomvals.Pnom/nomvals.w_Rnom;

elecparams.sigma = elecparams.L_S-(elecparams.M^2/elecparams.L_R);
elecparams.gamma = (elecparams.R_S*elecparams.L_R^2+elecparams.R_R*elecparams.M^2)/(elecparams.sigma*elecparams.L_R^2);

MI_params = struct('nomvals',nomvals,'elecparams',elecparams,'mechparams',mechparams);

== matlab function Modelo_MI_simulink_standalone_ver2020b/Inversor trifásico/Inversor 6 pulsos/Inversor/Calcular tiempos de conmutación/Angle to sector ==
  data: angle input; sector output
function sector = fcn(angle)

angle = angle*180/pi;

if angle >= 0 && angle <= 60
    sector = 1;
elseif angle > 60 && angle <= 120
    sector = 2;
elseif angle > 120 && angle <= 180
    sector = 3;
elseif angle > -180 && angle <= -120
    sector = 4;
elseif angle > -120 && angle <= -60
    sector = 5;
elseif angle > -60 && angle <= 0
    sector = 6;
else
    sector = -1;
end
